simulink model "Simulink_Gruppo_M"  (R2019b)
settings: Solver=VariableStepAuto  StartTime=0.0  StopTime=50  RelTol=1e-3
values from neighbouring files (symbols this model uses):
  A_n = 0.02    [Progetto_Gruppo_M.m]
  g = 6.67*(10^-11)    (= 6.67e-11)    [Progetto_Gruppo_M.m]
  I = 0.0075    [Progetto_Gruppo_M.m]
  Jp = 0.02    [Progetto_Gruppo_M.m]
  K = 3    [Progetto_Gruppo_M.m]
  L = 1    [Progetto_Gruppo_M.m]
  Mp = 0.07    [Progetto_Gruppo_M.m]
  ro = 0.2    [Progetto_Gruppo_M.m]
  u_ = Mp*g*L*sin(x_1r)    [Progetto_Gruppo_M.m]
  w_n = 100    [Progetto_Gruppo_M.m]
  wt = W*1    (= 5)    [Progetto_Gruppo_M.m]
  x_1g = 90    [Progetto_Gruppo_M.m]
  x_3 = (u_/K)+x_1g    [Progetto_Gruppo_M.m]
libraries: cstblocks x4, simulink_extras x2
settings Model: SimulationMode=accelerator  PacingRate=0.890000  Creator=ACER-aspire  LastModifiedBy=Filippo Manfreda
settings DataIOCC: ReturnWorkspaceOutputs=off
settings DebuggingCC: ArithmeticOperatorsInVariantConditions=warning
settings SFSimCC: SimUseLocalCustomCode=off  CustomCodeUndefinedFunction=UseInterfaceOnly
settings RTWCC: RTWUseLocalCustomCode=off

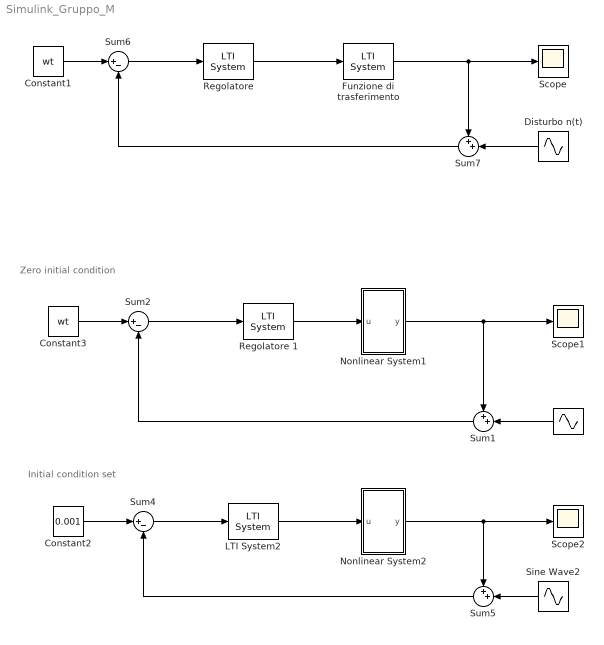
== system Simulink_Gruppo_M ==
  note: Initial condition set
  note: Zero initial condition
  " " : Sin  Amplitude=A_n  Frequency=w_n  SampleTime=0
  Constant1 : Constant  Value=wt
  Constant2 : Constant  Value=0.001
  Constant3 : Constant  Value=wt
  Disturbo n(t) : Sin  Amplitude=A_n  Frequency=w_n  SampleTime=0
  Funzione di trasferimento : cstblocks/LTI System  sys=G  IC=[]
  LTI System2 : cstblocks/LTI System  sys=R  IC=[]
  Nonlinear System1 : Subsystem
  Nonlinear System2 : Subsystem
  "Regolatore " : cstblocks/LTI System  sys=R  IC=[]
  Regolatore 1 : cstblocks/LTI System  sys=R  IC=[]
  "Scope " : Scope
  Scope1 : Scope
  Scope2 : Scope
  Sine Wave2 : Sin  Amplitude=0  Frequency=0  SampleTime=0
  Sum1 : Sum  Inputs=++|
  Sum2 : Sum  Inputs=|+-
  Sum4 : Sum  Inputs=|+-
  Sum5 : Sum  Inputs=++|
  Sum6 : Sum  Inputs=|+-
  Sum7 : Sum  Inputs=++|
  wires:
  Constant2/1 -> Sum4/1
  Sum4/1 -> LTI System2/1
  Nonlinear System2/1(y) -> Scope2/1, Sum5/1
  Sine Wave2/1 -> Sum5/2
  Sum5/1 -> Sum4/2
  "Regolatore "/1 -> Funzione di trasferimento/1
  Disturbo n(t)/1 -> Sum7/2
  Funzione di trasferimento/1 -> "Scope "/1, Sum7/1
  Sum6/1 -> "Regolatore "/1
  Sum7/1 -> Sum6/2
  Constant3/1 -> Sum2/1
  Constant1/1 -> Sum6/1
  Sum2/1 -> Regolatore 1/1
  Nonlinear System1/1(y) -> Sum1/1, Scope1/1
  Sum1/1 -> Sum2/2
  " "/1 -> Sum1/2
  Regolatore 1/1 -> Nonlinear System1/1(u)
  LTI System2/1 -> Nonlinear System2/1(u)

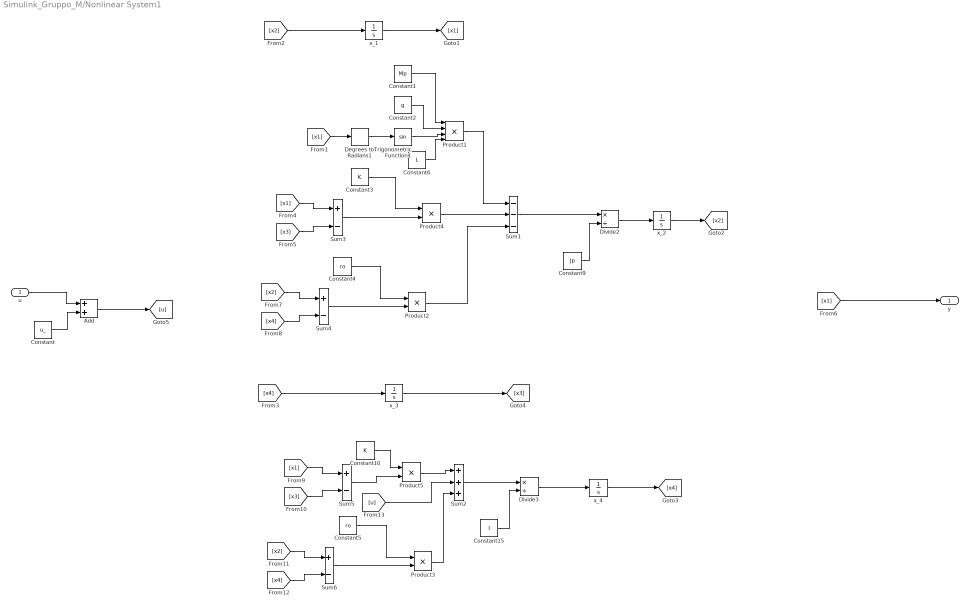
== system Simulink_Gruppo_M/Nonlinear System1 ==
  u : Inport
  Add : Sum
  Constant : Constant  Value=u_
  Constant1 : Constant  Value=Mp
  Constant10 : Constant  Value=K
  Constant15 : Constant  Value=I
  Constant2 : Constant  Value=g
  Constant3 : Constant  Value=K
  Constant4 : Constant  Value=ro
  Constant5 : Constant  Value=ro
  Constant6 : Constant  Value=L
  Constant9 : Constant  Value=Jp
  Degrees to Radians1 : simulink_extras/Transformations/Degrees to Radians
  Divide2 : Product  Inputs=*/
  Divide3 : Product  Inputs=*/
  Product1 : Product  Inputs=4
  Product{2..5} (4 alike) : Product
  Sum1 : Sum  Inputs=---
  Sum2 : Sum  Inputs=+++
  Sum{3..6} (4 alike) : Sum  Inputs=+-
  Trigonometric Function1 : Trigonometry
  x_1 : Integrator  InitialCondition=x_1g
  "x_2 " : Integrator
  x_3 : Integrator  InitialCondition=x_3
  x_4 : Integrator
  y : Outport  VectorParamsAs1DForOutWhenUnconnected=off
  wires:
  Constant9/1 -> Divide2/2
  Sum1/1 -> Divide2/1
  Divide2/1 -> "x_2 "/1
  "x_2 "/1 -> [x2]
  Constant10/1 -> Product5/1
  Product5/1 -> Sum2/1
  Sum2/1 -> Divide3/1
  Constant15/1 -> Divide3/2
  x_4/1 -> [x4]
  Divide3/1 -> x_4/1
  Trigonometric Function1/1 -> Product1/3
  [x1] -> Degrees to Radians1/1
  Degrees to Radians1/1 -> Trigonometric Function1/1
  Constant1/1 -> Product1/1
  Constant2/1 -> Product1/2
  Product4/1 -> Sum1/2
  Product1/1 -> Sum1/1
  [x2] -> x_1/1
  x_1/1 -> [x1]
  [x1] -> y/1
  [x4] -> x_3/1
  x_3/1 -> [x3]
  [x3] -> Sum3/2
  [x1] -> Sum3/1
  Sum3/1 -> Product4/2
  Constant3/1 -> Product4/1
  Sum4/1 -> Product2/2
  Constant4/1 -> Product2/1
  [x2] -> Sum4/1
  [x4] -> Sum4/2
  Product2/1 -> Sum1/3
  [x1] -> Sum5/1
  [x3] -> Sum5/2
  Sum5/1 -> Product5/2
  Sum6/1 -> Product3/2
  [x4] -> Sum6/2
  Constant5/1 -> Product3/1
  [x2] -> Sum6/1
  Product3/1 -> Sum2/3
  Constant6/1 -> Product1/4
  Constant/1 -> Add/2
  u/1 -> Add/1
  Add/1 -> [u]
  [u] -> Sum2/2

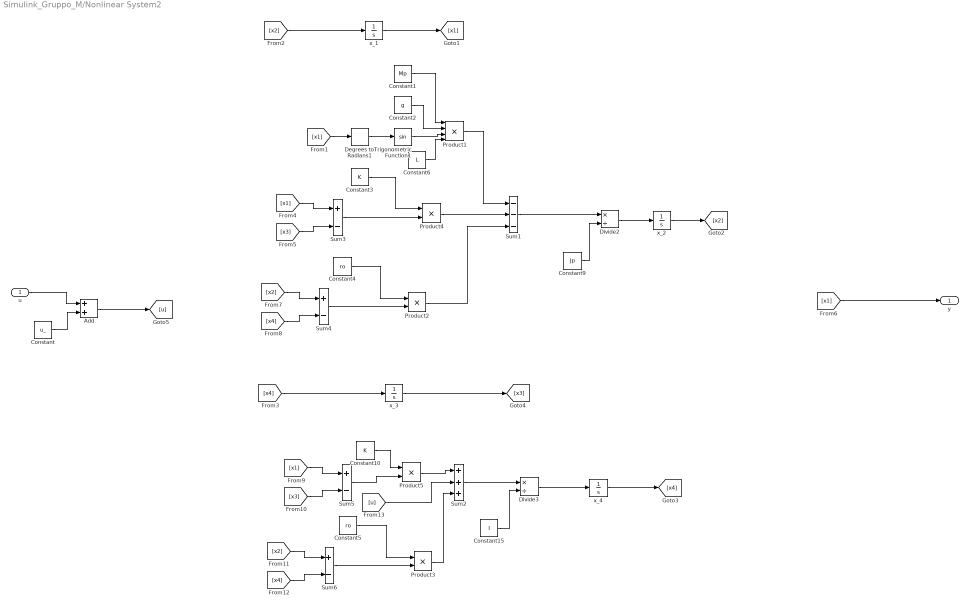
== system Simulink_Gruppo_M/Nonlinear System2 ==
  u : Inport
  Add : Sum
  Constant : Constant  Value=u_
  Constant1 : Constant  Value=Mp
  Constant10 : Constant  Value=K
  Constant15 : Constant  Value=I
  Constant2 : Constant  Value=g
  Constant3 : Constant  Value=K
  Constant4 : Constant  Value=ro
  Constant5 : Constant  Value=ro
  Constant6 : Constant  Value=L
  Constant9 : Constant  Value=Jp
  Degrees to Radians1 : simulink_extras/Transformations/Degrees to Radians
  Divide2 : Product  Inputs=*/
  Divide3 : Product  Inputs=*/
  Product1 : Product  Inputs=4
  Product{2..5} (4 alike) : Product
  Sum1 : Sum  Inputs=---
  Sum2 : Sum  Inputs=+++
  Sum{3..6} (4 alike) : Sum  Inputs=+-
  Trigonometric Function1 : Trigonometry
  x_1 : Integrator  InitialCondition=x_1g
  "x_2 " : Integrator
  x_3 : Integrator  InitialCondition=x_3
  x_4 : Integrator
  y : Outport  VectorParamsAs1DForOutWhenUnconnected=off
  wires:
  Constant9/1 -> Divide2/2
  Sum1/1 -> Divide2/1
  Divide2/1 -> "x_2 "/1
  "x_2 "/1 -> [x2]
  Constant10/1 -> Product5/1
  Product5/1 -> Sum2/1
  Sum2/1 -> Divide3/1
  Constant15/1 -> Divide3/2
  x_4/1 -> [x4]
  Divide3/1 -> x_4/1
  Trigonometric Function1/1 -> Product1/3
  [x1] -> Degrees to Radians1/1
  Degrees to Radians1/1 -> Trigonometric Function1/1
  Constant1/1 -> Product1/1
  Constant2/1 -> Product1/2
  Product4/1 -> Sum1/2
  Product1/1 -> Sum1/1
  [x2] -> x_1/1
  x_1/1 -> [x1]
  [x1] -> y/1
  [x4] -> x_3/1
  x_3/1 -> [x3]
  [x3] -> Sum3/2
  [x1] -> Sum3/1
  Sum3/1 -> Product4/2
  Constant3/1 -> Product4/1
  Sum4/1 -> Product2/2
  Constant4/1 -> Product2/1
  [x2] -> Sum4/1
  [x4] -> Sum4/2
  Product2/1 -> Sum1/3
  [x1] -> Sum5/1
  [x3] -> Sum5/2
  Sum5/1 -> Product5/2
  Sum6/1 -> Product3/2
  [x4] -> Sum6/2
  Constant5/1 -> Product3/1
  [x2] -> Sum6/1
  Product3/1 -> Sum2/3
  Constant6/1 -> Product1/4
  Constant/1 -> Add/2
  u/1 -> Add/1
  Add/1 -> [u]
  [u] -> Sum2/2
